simulink model "Rooms_integrated_bus13"  (R2025a)
settings: Solver=VariableStepAuto  StartTime=0.0  StopTime=5  RelTol=1e-3
libraries: spsThreePhaseVIMeasurementLib x53, fl_lib x40, nesl_utility x24, spsThreePhaseSeriesRLCLoadLib x20, spsThreePhasePISectionLineLib x20, spsLoadFlowBusLib x19, simulink x8, spsThreePhaseBreakerLib x8, spspowerguiLib x8, spsThreePhaseTransformerTwoWindingsLib x5, spsThreePhaseSourceLib x5, sps_lib x1
(part 3 of 4)

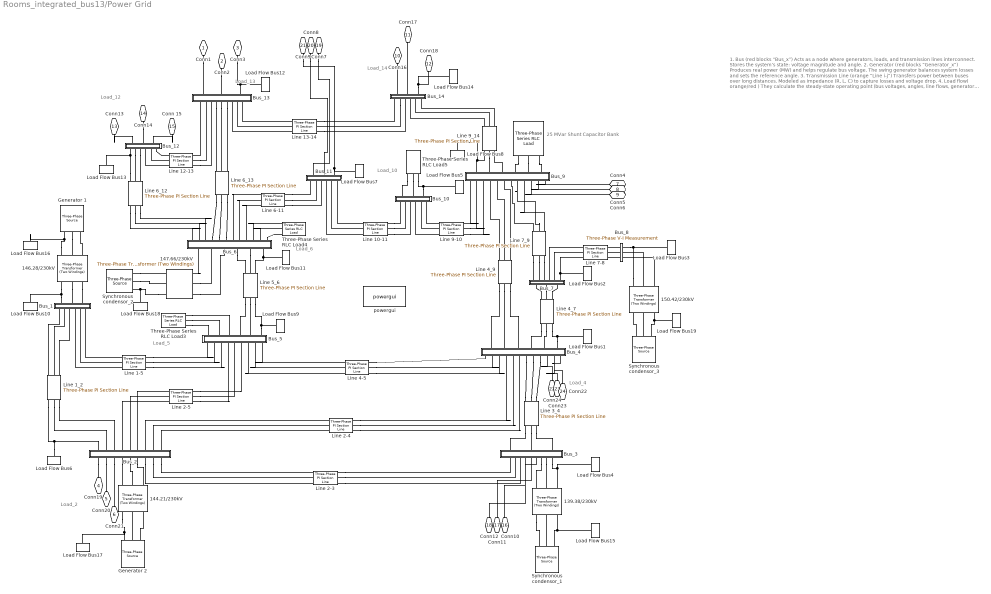
== system Rooms_integrated_bus13/Power Grid ==
  note: 1. Bus (red blocks “Bus_x”)
      | Acts as a node where generators, loads, and transmission lines interconnect.
      | Stores the system’s state: voltage magnitude and angle.
      | 2. Generator (red blocks “Generator_x”)
      | Produces real power (MW) and helps regulate bus voltage.
      | The swing generator balances system losses and sets the reference angle.
      | 3. Transmission Line (orange “Line i-j”)
      | Transfers power between buses over long distances.
      | Modeled as impedance (R, L, C) to capture losses and voltage drop.
      | 4. Load flow( orange/red )
      | They calculate the steady-state operating point (bus voltages, angles, line flows, generator outputs) before starting the simulation.
      | They provide the initial pu values (e.g., voltage magnitude & angle at each bus) so the dynamic model starts from a realistic balanced condition. .
      | 5. Synchronous Condenser (red blocks)
      | A synchronous machine running without mechanical load.
      | Supplies or absorbs reactive power to support voltage stability.
      | 6. Shunt Capacitor Bank
      | Provides fixed reactive power (Q) compensation.
      | Improves voltage profile and reduces reactive power flow in lines.
      | 7. Custom Connection Blocks (Conn1, Conn2, …)
      | Interfaces to external/custom subsystems instead of static loads.
      | Allow modeling of dynamic or special loads (e.g., EVs, converters, FACTS).
      | .
  note: Load_5
  note: Load_13
  note: Load_6
  note: Load_10
  note: Load_12
  note: Load_14
  note: Load_4
  note: 25 MVar Shunt
      | Capacitor Bank
  note: Load_2
  " " : spsThreePhaseSeriesRLCLoadLib/Three-Phase Series RLC Load  LConnTagsString=A|B|C  Configuration=Y (grounded)  NominalVoltage=230e3  Vabc=[1e3 1e3 1e3]  Vabcp=[1e3 1e3 1e3]  NominalFrequency=60  UnbalancedPower=off  ActivePower=0  InductivePower=0  CapacitivePower=25e6  Pabc=[10e3 9e3 11e3]  QLabc=[100 90 110]  QCabc=[100 90 110]  Pabcp=[10e3 9e3 11e3]  QLabcp=[100 90 110]  QCabcp=[100 90 110]  Measurements=None  LoadType=constant Z
  139.38/230kV : spsThreePhaseTransformerTwoWindingsLib/Three-Phase Transformer (Two Windings)  Winding1Connection=Yg  Winding2Connection=Yg  CoreType=Three single-phase transformers  SetSaturation=off  Hysteresis=off  DataFile='hysteresis'  SetInitialFlux=off  Measurements=None  UNITS=pu  NominalPower=[ 120e6 , 60 ]  Winding1=[139.38e3 , 0.002 , 0.08 ]  Winding2=[ 230e3 , 0.002 , 0.08 ]  Rm=500  Lm=500  L0=0.5  Saturation=[ 0,0 ; 0.0024,1.2 ; 1.0,1.52 ]  InitialFluxes=[ 0.8 , -0.8 , 0.7 ]  BreakLoop=off  DiscreteSolver=Trapezoidal iterative  DataType=off  TransfoNumber=1
  144.21/230kV : spsThreePhaseTransformerTwoWindingsLib/Three-Phase Transformer (Two Windings)  Winding1Connection=Yg  Winding2Connection=Yg  CoreType=Three single-phase transformers  SetSaturation=off  Hysteresis=off  DataFile='hysteresis'  SetInitialFlux=off  Measurements=None  UNITS=pu  NominalPower=[ 120e6 , 60 ]  Winding1=[144.21e3 , 0.002 , 0.08 ]  Winding2=[ 230e3 , 0.002 , 0.08 ]  Rm=500  Lm=500  L0=0.5  Saturation=[ 0,0 ; 0.0024,1.2 ; 1.0,1.52 ]  InitialFluxes=[ 0.8 , -0.8 , 0.7 ]  BreakLoop=off  DiscreteSolver=Trapezoidal iterative  DataType=off  TransfoNumber=1
  146.28/230kV : spsThreePhaseTransformerTwoWindingsLib/Three-Phase Transformer (Two Windings)  Winding1Connection=Yg  Winding2Connection=Yg  CoreType=Three single-phase transformers  SetSaturation=off  Hysteresis=off  DataFile='hysteresis'  SetInitialFlux=off  Measurements=None  UNITS=pu  NominalPower=[ 120e6 , 60 ]  Winding1=[146.28e3 , 0.002 , 0.08 ]  Winding2=[ 230e3 , 0.002 , 0.08 ]  Rm=500  Lm=500  L0=0.5  Saturation=[ 0,0 ; 0.0024,1.2 ; 1.0,1.52 ]  InitialFluxes=[ 0.8 , -0.8 , 0.7 ]  BreakLoop=off  DiscreteSolver=Trapezoidal iterative  DataType=off  TransfoNumber=1
  147.66/230kV : spsThreePhaseTransformerTwoWindingsLib/Three-Phase Transformer (Two Windings)  Winding1Connection=Yg  Winding2Connection=Yg  CoreType=Three single-phase transformers  SetSaturation=off  Hysteresis=off  DataFile='hysteresis'  SetInitialFlux=off  Measurements=None  UNITS=pu  NominalPower=[ 120e6 , 60 ]  Winding1=[147.66e3 , 0.002 , 0.08 ]  Winding2=[ 230e3 , 0.002 , 0.08 ]  Rm=500  Lm=500  L0=0.5  Saturation=[ 0,0 ; 0.0024,1.2 ; 1.0,1.52 ]  InitialFluxes=[ 0.8 , -0.8 , 0.7 ]  BreakLoop=off  DiscreteSolver=Trapezoidal iterative  DataType=off  TransfoNumber=1
  150.42/230kV : spsThreePhaseTransformerTwoWindingsLib/Three-Phase Transformer (Two Windings)  Winding1Connection=Yg  Winding2Connection=Yg  CoreType=Three single-phase transformers  SetSaturation=off  Hysteresis=off  DataFile='hysteresis'  SetInitialFlux=off  Measurements=None  UNITS=pu  NominalPower=[ 120e6 , 60 ]  Winding1=[150.42e3 , 0.002 , 0.08 ]  Winding2=[ 230e3 , 0.002 , 0.08 ]  Rm=500  Lm=500  L0=0.5  Saturation=[ 0,0 ; 0.0024,1.2 ; 1.0,1.52 ]  InitialFluxes=[ 0.8 , -0.8 , 0.7 ]  BreakLoop=off  DiscreteSolver=Trapezoidal iterative  DataType=off  TransfoNumber=1
  Bus_1 : Subsystem
  Bus_10 : Subsystem
  Bus_11 : Subsystem
  Bus_12 : Subsystem
  Bus_13 : Subsystem
  Bus_14 : Subsystem
  Bus_2 : Subsystem
  Bus_3 : Subsystem
  Bus_4 : Subsystem
  Bus_5 : Subsystem
  Bus_6 : Subsystem
  Bus_7 : Subsystem
  Bus_8 : spsThreePhaseVIMeasurementLib/Three-Phase V-I Measurement  VoltageMeasurement=phase-to-phase  SetLabelV=on  LabelV=VB_8  Vpu=off  VpuLL=off  CurrentMeasurement=yes  SetLabelI=on  LabelI=IB_8  Ipu=off  Pbase=100e6  Vbase=500e3  OutputType=Complex  PhasorSimulation=off  PSBequivalent=0
  Bus_9 : Subsystem
  Generator 1 : spsThreePhaseSourceLib/Three-Phase Source  InternalConnection=Yg  VoltagePhases=off  Voltage=(146280)*1.03071  PhaseAngle=3.7708  Voltage_phases=[25e3 25e3 25e3]/sqrt(3)  PhaseAngles_phases=[0 -120 +120]  Frequency=60  NonIdealSource=on  SpecifyImpedance=off  Resistance=0.8929  Inductance=16.58e-3  ShortCircuitLevel=100e6  BaseVoltage=146.28e3  XRratio=7  BusType=swing  Pref=163e6  Qref=0  Prefabc=[10e3, 10e3, 10e3]  Qrefabc=[0, 0, 0]  Qmin=-inf  Qmax=inf
  Generator 2 : spsThreePhaseSourceLib/Three-Phase Source  InternalConnection=Yg  VoltagePhases=off  Voltage=(144210)*1.01655  PhaseAngle=-15.8323  Voltage_phases=[25e3 25e3 25e3]/sqrt(3)  PhaseAngles_phases=[0 -120 +120]  Frequency=60  NonIdealSource=on  SpecifyImpedance=off  Resistance=0.8929  Inductance=16.58e-3  ShortCircuitLevel=100e6  BaseVoltage=144.21e3  XRratio=7  BusType=PV  Pref=90e6  Qref=0  Prefabc=[10e3, 10e3, 10e3]  Qrefabc=[0, 0, 0]  Qmin=-inf  Qmax=inf
  Line 1-5 : spsThreePhasePISectionLineLib/Three-Phase PI Section Line  LConnTagsString=a|b|c  RConnTagsString=A|B|C  Length=78.64  Frequency=60  Resistances=[ 0.3029 0.9086]  Inductances=[ 0.0033 0.0099]  Capacitances=[3.35e-9 1.01e-8]
  Line 10-11 : spsThreePhasePISectionLineLib/Three-Phase PI Section Line  LConnTagsString=a|b|c  RConnTagsString=A|B|C  Length=4.93  Frequency=60  Resistances=[ 0.3667 1.1002]  Inductances=[ 0.0023 0.0068]  Capacitances=[1.22e-11 3.66e-11]
  Line 12-13 : spsThreePhasePISectionLineLib/Three-Phase PI Section Line  LConnTagsString=a|b|c  RConnTagsString=A|B|C  Length=5.03  Frequency=60  Resistances=[ 0.9679 2.9038]  Inductances=[ 0.0023 0.0070]  Capacitances=[1.20e-11 3.59e-11]
  Line 13-14 : spsThreePhasePISectionLineLib/Three-Phase PI Section Line  LConnTagsString=a|b|c  RConnTagsString=A|B|C  Length=6.64  Frequency=60  Resistances=[ 0.5676 1.7027]  Inductances=[ 0.0031 0.0092]  Capacitances=[9.06e-12 2.72e-11]
  Line 1_2 : spsThreePhasePISectionLineLib/Three-Phase PI Section Line  LConnTagsString=a|b|c  RConnTagsString=A|B|C  Length=44.47  Frequency=60  Resistances=[ 0.1921 0.5763]  Inductances=[ 0.0016 0.0047]  Capacitances=[7.14e-9 2.14e-8]
  Line 2-3 : spsThreePhasePISectionLineLib/Three-Phase PI Section Line  LConnTagsString=a|b|c  RConnTagsString=A|B|C  Length=68.47  Frequency=60  Resistances=[ 0.3026 0.9077]  Inductances=[ 0.0034 0.0101]  Capacitances=[3.29e-9 9.86e-8]
  Line 2-4 : spsThreePhasePISectionLineLib/Three-Phase PI Section Line  LConnTagsString=a|b|c  RConnTagsString=A|B|C  Length=74.11  Frequency=60  Resistances=[ 0.3457 1.0370]  Inductances=[ 0.0028 0.0083]  Capacitances=[3.99e-9 1.20e-8]
  Line 2-5 : spsThreePhasePISectionLineLib/Three-Phase PI Section Line  LConnTagsString=a|b|c  RConnTagsString=A|B|C  Length=61.18  Frequency=60  Resistances=[ 0.4104 1.2311]  Inductances=[ 0.0033 0.0100]  Capacitances=[3.34e-9 1.0e-8]
  Line 3_4 : spsThreePhasePISectionLineLib/Three-Phase PI Section Line  LConnTagsString=a|b|c  RConnTagsString=A|B|C  Length=61.21  Frequency=60  Resistances=[ 0.4826 1.4479]  Inductances=[ 0.0033 0.0098]  Capacitances=[3.4e-9 1.02e-8]
  Line 4-5 : spsThreePhasePISectionLineLib/Three-Phase PI Section Line  LConnTagsString=a|b|c  RConnTagsString=A|B|C  Length=18.47  Frequency=60  Resistances=[ 0.3186 0.9558]  Inductances=[ 0.0027 0.0080]  Capacitances=[4.17e-9 1.25e-8]
  Line 4_7 : spsThreePhasePISectionLineLib/Three-Phase PI Section Line  LConnTagsString=a|b|c  RConnTagsString=A|B|C  Length=5.15  Frequency=60  Resistances=[ 0.0001 0.0003]  Inductances=[ 0.0475 0.1425]  Capacitances=[2.34e-10 7.02e-10]
  Line 4_9 : spsThreePhasePISectionLineLib/Three-Phase PI Section Line  LConnTagsString=a|b|c  RConnTagsString=A|B|C  Length=8.39  Frequency=60  Resistances=[ 0.0001 0.0003]  Inductances=[ 0.0775 0.2325]  Capacitances=[1.43e-10 4.3e-10]
  Line 5_6 : spsThreePhasePISectionLineLib/Three-Phase PI Section Line  LConnTagsString=a|b|c  RConnTagsString=A|B|C  Length=5.65  Frequency=60  Resistances=[ 0.0001 0.0003]  Inductances=[ 0.0522 0.1565]  Capacitances=[2.13e-10 6.39e-10]
  Line 6-11 : spsThreePhasePISectionLineLib/Three-Phase PI Section Line  LConnTagsString=a|b|c  RConnTagsString=A|B|C  Length=5.02  Frequency=60  Resistances=[ 0.4172 1.2515]  Inductances=[ 0.0023 0.0070]  Capacitances=[1.20e-11 3.60e-11]
  Line 6_12 : spsThreePhasePISectionLineLib/Three-Phase PI Section Line  LConnTagsString=a|b|c  RConnTagsString=A|B|C  Length=5.69  Frequency=60  Resistances=[ 0.4760 1.4281]  Inductances=[ 0.0026 0.0079]  Capacitances=[1.06e-11 3.17e-11]
  Line 6_13 : spsThreePhasePISectionLineLib/Three-Phase PI Section Line  LConnTagsString=a|b|c  RConnTagsString=A|B|C  Length=4.06  Frequency=60  Resistances=[ 0.3590 1.0770]  Inductances=[ 0.0019 0.0056]  Capacitances=[1.48e-11 4.44e-11]
  Line 7-8 : spsThreePhasePISectionLineLib/Three-Phase PI Section Line  LConnTagsString=a|b|c  RConnTagsString=A|B|C  Length=4.72  Frequency=60  Resistances=[ 0.0005 0.0014]  Inductances=[ 0.0022 0.0065]  Capacitances=[ 1.27e-11 3.82e-11]
  Line 7_9 : spsThreePhasePISectionLineLib/Three-Phase PI Section Line  LConnTagsString=a|b|c  RConnTagsString=A|B|C  Length=3.73  Frequency=60  Resistances=[ 0.0006 0.0018]  Inductances=[ 0.0017 0.0052]  Capacitances=[ 1.61e-11 4.84e-11]
  Line 9-10 : spsThreePhasePISectionLineLib/Three-Phase PI Section Line  LConnTagsString=a|b|c  RConnTagsString=A|B|C  Length=3.27  Frequency=60  Resistances=[ 0.2144 0.6431]  Inductances=[ 0.0015 0.0045]  Capacitances=[1.84e-11 5.52e-11]
  Line 9_14 : spsThreePhasePISectionLineLib/Three-Phase PI Section Line  LConnTagsString=a|b|c  RConnTagsString=A|B|C  Length=5.85  Frequency=60  Resistances=[ 0.4788 1.4365]  Inductances=[ 0.0027 0.0081]  Capacitances=[1.03e-11 3.08e-11]
  Load Flow Bus1 : spsLoadFlowBusLib/Load Flow Bus  LConnTagsString=a  Phases=single  Connectors=on one side  ID=BUS_4  Vbase=230e3  Vref=1  Vangle=0  VLF=0.928  VLFb=1  VLFc=1  angleLF=-31.28  angleLFb=0  angleLFc=0
  Load Flow Bus10 : spsLoadFlowBusLib/Load Flow Bus  LConnTagsString=a  Phases=single  Connectors=on one side  ID=BUS_1  Vbase=230e3  Vref=1.0  Vangle=0  VLF=0.9625  VLFb=1  VLFc=1  angleLF=-19.37  angleLFb=0  angleLFc=0
  Load Flow Bus11 : spsLoadFlowBusLib/Load Flow Bus  LConnTagsString=a  Phases=single  Connectors=on one side  ID=BUS_6  Vbase=230e3  Vref=1  Vangle=0  VLF=0.9425  VLFb=1  VLFc=1  angleLF=-36.08  angleLFb=0  angleLFc=0
  Load Flow Bus12 : spsLoadFlowBusLib/Load Flow Bus  LConnTagsString=a  Phases=single  Connectors=on one side  ID=BUS_13  Vbase=230e3  Vref=1  Vangle=0  VLF=0.9416  VLFb=1  VLFc=1  angleLF=-36.14  angleLFb=0  angleLFc=0
  Load Flow Bus13 : spsLoadFlowBusLib/Load Flow Bus  LConnTagsString=a  Phases=single  Connectors=on one side  ID=BUS_12  Vbase=230e3  Vref=1.0  Vangle=0  VLF=0.9418  VLFb=1  VLFc=1  angleLF=-36.13  angleLFb=0  angleLFc=0
  Load Flow Bus14 : spsLoadFlowBusLib/Load Flow Bus  LConnTagsString=a  Phases=single  Connectors=on one side  ID=BUS_14  Vbase=230e3  Vref=1  Vangle=0  VLF=0.9414  VLFb=1  VLFc=1  angleLF=-36.19  angleLFb=0  angleLFc=0
  Load Flow Bus15 : spsLoadFlowBusLib/Load Flow Bus  LConnTagsString=a  Phases=single  Connectors=on one side  ID=BUS_c  Vbase=139.38e3  Vref=1  Vangle=0  VLF=0.9282  VLFb=1  VLFc=1  angleLF=-34.24  angleLFb=0  angleLFc=0
  Load Flow Bus16 : spsLoadFlowBusLib/Load Flow Bus  LConnTagsString=a  Phases=single  Connectors=on one side  ID=BUS_a  Vbase=146.28e3  Vref=1.0  Vangle=0  VLF=0.9625  VLFb=1  VLFc=1  angleLF=-19.37  angleLFb=0  angleLFc=0
  Load Flow Bus17 : spsLoadFlowBusLib/Load Flow Bus  LConnTagsString=a  Phases=single  Connectors=on one side  ID=BUS_b  Vbase=144.21e3  Vref=1.025  Vangle=0  VLF=0.9497  VLFb=1  VLFc=1  angleLF=-24.42  angleLFb=0  angleLFc=0
  Load Flow Bus18 : spsLoadFlowBusLib/Load Flow Bus  LConnTagsString=a  Phases=single  Connectors=on one side  ID=BUS_d  Vbase=147.66e3  Vref=1.0  Vangle=0  VLF=0.9625  VLFb=1  VLFc=1  angleLF=-19.37  angleLFb=0  angleLFc=0
  Load Flow Bus19 : spsLoadFlowBusLib/Load Flow Bus  LConnTagsString=a  Phases=single  Connectors=on one side  ID=BUS_e  Vbase=150.420e3  Vref=1  Vangle=0  VLF=0.9461  VLFb=1  VLFc=1  angleLF=-36  angleLFb=0  angleLFc=0
  Load Flow Bus2 : spsLoadFlowBusLib/Load Flow Bus  LConnTagsString=a  Phases=single  Connectors=on one side  ID=BUS_7  Vbase=230e3  Vref=1  Vangle=0  VLF=0.9439  VLFb=1  VLFc=1  angleLF=-36  angleLFb=0  angleLFc=0
  Load Flow Bus3 : spsLoadFlowBusLib/Load Flow Bus  LConnTagsString=a  Phases=single  Connectors=on one side  ID=BUS_8  Vbase=230e3  Vref=1  Vangle=0  VLF=0.9461  VLFb=1  VLFc=1  angleLF=-36  angleLFb=0  angleLFc=0
  Load Flow Bus4 : spsLoadFlowBusLib/Load Flow Bus  LConnTagsString=a  Phases=single  Connectors=on one side  ID=BUS_3  Vbase=230e3  Vref=1  Vangle=0  VLF=0.9282  VLFb=1  VLFc=1  angleLF=-34.24  angleLFb=0  angleLFc=0
  Load Flow Bus5 : spsLoadFlowBusLib/Load Flow Bus  LConnTagsString=a  Phases=single  Connectors=on one side  ID=BUS_10  Vbase=230e3  Vref=1  Vangle=0  VLF=0.9425  VLFb=1  VLFc=1  angleLF=-36.13  angleLFb=0  angleLFc=0
  Load Flow Bus6 : spsLoadFlowBusLib/Load Flow Bus  LConnTagsString=a  Phases=single  Connectors=on one side  ID=BUS_2  Vbase=230e3  Vref=1.0  Vangle=0  VLF=0.9497  VLFb=1  VLFc=1  angleLF=-24.42  angleLFb=0  angleLFc=0
  Load Flow Bus7 : spsLoadFlowBusLib/Load Flow Bus  LConnTagsString=a  Phases=single  Connectors=on one side  ID=BUS_11  Vbase=230e3  Vref=1  Vangle=0  VLF=0.9423  VLFb=1  VLFc=1  angleLF=-36.11  angleLFb=0  angleLFc=0
  Load Flow Bus8 : spsLoadFlowBusLib/Load Flow Bus  LConnTagsString=a  Phases=single  Connectors=on one side  ID=BUS_9  Vbase=230e3  Vref=1.0  Vangle=0  VLF=0.943  VLFb=1  VLFc=1  angleLF=-36.12  angleLFb=0  angleLFc=0
  Load Flow Bus9 : spsLoadFlowBusLib/Load Flow Bus  LConnTagsString=a  Phases=single  Connectors=on one side  ID=BUS_5  Vbase=230e3  Vref=1  Vangle=0  VLF=0.9312  VLFb=1  VLFc=1  angleLF=-29.41  angleLFb=0  angleLFc=0
  Synchronous condensor_1 : spsThreePhaseSourceLib/Three-Phase Source  InternalConnection=Yg  VoltagePhases=off  Voltage=(139380)*1.01137  PhaseAngle=-34.48  Voltage_phases=[25e3 25e3 25e3]/sqrt(3)  PhaseAngles_phases=[0 -120 +120]  Frequency=60  NonIdealSource=on  SpecifyImpedance=off  Resistance=0.8929  Inductance=16.58e-3  ShortCircuitLevel=100e6  BaseVoltage=139.38e3  XRratio=7  BusType=PQ  Pref=0  Qref=50.096e6  Prefabc=[10e3, 10e3, 10e3]  Qrefabc=[0, 0, 0]  Qmin=-inf  Qmax=inf
  Synchronous condensor_2 : spsThreePhaseSourceLib/Three-Phase Source  InternalConnection=Yg  VoltagePhases=off  Voltage=(147660)*0.984306  PhaseAngle=-36.2022  Voltage_phases=[25e3 25e3 25e3]/sqrt(3)  PhaseAngles_phases=[0 -120 +120]  Frequency=60  NonIdealSource=on  SpecifyImpedance=off  Resistance=0.8929  Inductance=16.58e-3  ShortCircuitLevel=100e6  BaseVoltage=147.66e3  XRratio=7  BusType=PQ  Pref=0  Qref=25.276e6  Prefabc=[10e3, 10e3, 10e3]  Qrefabc=[0, 0, 0]  Qmin=-inf  Qmax=inf
  Synchronous condensor_3 : spsThreePhaseSourceLib/Three-Phase Source  InternalConnection=Yg  VoltagePhases=off  Voltage=(150420)*0.995122  PhaseAngle=-36.1424  Voltage_phases=[25e3 25e3 25e3]/sqrt(3)  PhaseAngles_phases=[0 -120 +120]  Frequency=60  NonIdealSource=on  SpecifyImpedance=off  Resistance=0.8929  Inductance=16.58e-3  ShortCircuitLevel=100e6  BaseVoltage=150.42e3  XRratio=7  BusType=PQ  Pref=0  Qref=30.144e6  Prefabc=[10e3, 10e3, 10e3]  Qrefabc=[0, 0, 0]  Qmin=-inf  Qmax=inf
  Three-Phase Series RLC Load3 : spsThreePhaseSeriesRLCLoadLib/Three-Phase Series RLC Load  LConnTagsString=A|B|C  Configuration=Y (grounded)  NominalVoltage=(230000)*0.931217  Vabc=[1e3 1e3 1e3]  Vabcp=[1e3 1e3 1e3]  NominalFrequency=60  UnbalancedPower=off  ActivePower=9.12e6  InductivePower=1.92e6  CapacitivePower=0  Pabc=[10e3 9e3 11e3]  QLabc=[100 90 110]  QCabc=[100 90 110]  Pabcp=[10e3 9e3 11e3]  QLabcp=[100 90 110]  QCabcp=[100 90 110]  Measurements=None  LoadType=constant PQ
  Three-Phase Series RLC Load4 : spsThreePhaseSeriesRLCLoadLib/Three-Phase Series RLC Load  LConnTagsString=A|B|C  Configuration=Y (grounded)  NominalVoltage=(230000)*0.942548  Vabc=[1e3 1e3 1e3]  Vabcp=[1e3 1e3 1e3]  NominalFrequency=60  UnbalancedPower=off  ActivePower=13.44e6  InductivePower=9e6  CapacitivePower=0  Pabc=[10e3 9e3 11e3]  QLabc=[100 90 110]  QCabc=[100 90 110]  Pabcp=[10e3 9e3 11e3]  QLabcp=[100 90 110]  QCabcp=[100 90 110]  Measurements=None  LoadType=constant PQ
  Three-Phase Series RLC Load5 : spsThreePhaseSeriesRLCLoadLib/Three-Phase Series RLC Load  LConnTagsString=A|B|C  Configuration=Y (grounded)  NominalVoltage=(230000)*0.942502  Vabc=[1e3 1e3 1e3]  Vabcp=[1e3 1e3 1e3]  NominalFrequency=60  UnbalancedPower=off  ActivePower=10.8e6  InductivePower=6.96e6  CapacitivePower=0  Pabc=[10e3 9e3 11e3]  QLabc=[100 90 110]  QCabc=[100 90 110]  Pabcp=[10e3 9e3 11e3]  QLabcp=[100 90 110]  QCabcp=[100 90 110]  Measurements=None  LoadType=constant PQ
  powergui : spspowerguiLib/powergui  Priority=1  SimulationMode=Discrete  SampleTime=50e-6  frequency=60  Iterations=50  frequencyindice=60  Pbase=120e6  ErrMax=0.0001  UnitsV=kV  UnitsW=MW  buscounter=0  FunctionMessages=off  echomessages=off  EnableUseOfTLC=off  CurrentSourceSwitches=off  DisableSnubberDevices=off  DisableRonSwitches=off  DisableVfSwitches=off  DisplayEquations=off  AutomaticDiscreteSolvers=off  SolverType=Tustin/Backward Euler (TBE)  Interpol=off  ExternalGateDelay=off  methode=off  Ts=100  x0status=blocks  SPID=on  SwTol=0  HookPort=off  NonlinearTolerance=1e-4  nMaxIteration=100  ContinueOnMaxIteration=off  RestoreLinks=warning  ResistiveCurrentMeasurement=off  Frange=[0:2:500]  Ylog=off  Xlog=on  ShowGrid=off  save=off  variable=ZData  structure=0  ZoomFFT=off  StartTime=0.0  cycles=1  DisplayStyle=1  fundamental=60  FreqAxis=off  MaxFrequency=1000  frequencyindicesteady=1  RmsSteady=1  display=off
  Conn1 : PMIOPort  Side=Left
  Conn2 : PMIOPort  Port=2  Side=Left
  Conn3 : PMIOPort  Port=3  Side=Left
  Conn19 : PMIOPort  Port=4  Side=Left
  Conn20 : PMIOPort  Port=5  Side=Left
  Conn21 : PMIOPort  Port=6  Side=Left
  Conn4 : PMIOPort  Port=7  Side=Left
  Conn5 : PMIOPort  Port=8  Side=Left
  Conn6 : PMIOPort  Port=9  Side=Left
  Conn16 : PMIOPort  Port=10  Side=Left
  Conn17 : PMIOPort  Port=11  Side=Left
  Conn18 : PMIOPort  Port=12  Side=Left
  Conn13 : PMIOPort  Port=13  Side=Right
  Conn14 : PMIOPort  Port=14  Side=Right
  Conn 15 : PMIOPort  Port=15  Side=Right
  Conn10 : PMIOPort  Port=16  Side=Right
  Conn11 : PMIOPort  Port=17  Side=Right
  Conn12 : PMIOPort  Port=18  Side=Right
  Conn7 : PMIOPort  Port=19  Side=Right
  Conn8 : PMIOPort  Port=20  Side=Right
  Conn9 : PMIOPort  Port=21  Side=Right
  Conn24 : PMIOPort  Port=22  Side=Right
  Conn23 : PMIOPort  Port=23  Side=Right
  Conn22 : PMIOPort  Port=24  Side=Right
  connections:
  Synchronous condensor_3/RConn1 -- 150.42/230kV/LConn1
  Bus_2/RConn4 -- 144.21/230kV/RConn1
  Line 10-11/LConn1 -- Bus_11/RConn6
  Line 6_12/RConn1 -- Bus_6/RConn1
  147.66/230kV/LConn3 -- Synchronous condensor_2/RConn3 -- Load Flow Bus18/LConn1
  Line 2-5/RConn3 -- Bus_5/RConn4
  Conn7/RConn1 -- Bus_11/LConn1
  Line 9_14/RConn1 -- Bus_9/LConn1 -- Load Flow Bus8/LConn1
  Bus_4/RConn7 -- Line 3_4/LConn1
  146.28/230kV/RConn1 -- Bus_1/LConn3
  Line 12-13/RConn3 -- Bus_13/RConn3
  Line 9-10/LConn3 -- Bus_10/RConn4
  Line 2-5/RConn2 -- Bus_5/RConn5
  Generator 2/RConn1 -- 144.21/230kV/LConn1 -- Load Flow Bus17/LConn1
  Line 4_9/RConn1 -- Bus_4/LConn1
  Bus_2/LConn5 -- Line 2-5/LConn2
  Load Flow Bus12/LConn1 -- Conn3/RConn1 -- Bus_13/LConn3
  Bus_5/LConn6 -- Line 5_6/RConn3 -- Load Flow Bus9/LConn1
  Load Flow Bus11/LConn1 -- Bus_6/LConn6 -- Line 5_6/LConn3
  Bus_11/LConn3 -- Conn9/RConn1 -- Load Flow Bus7/LConn1
  147.66/230kV/RConn3 -- Bus_6/LConn3
  Line 4_7/RConn1 -- Bus_4/LConn4
  Line 4-5/RConn1 -- Bus_4/RConn1
  Bus_6/LConn5 -- Line 5_6/LConn2
  Bus_14/LConn3 -- Conn18/RConn1 -- Load Flow Bus14/LConn1
  Line 9-10/RConn2 -- Bus_9/RConn2
  Line 6-11/RConn2 -- Bus_11/RConn2
  Line 4-5/LConn2 -- Bus_5/RConn8
  Bus_2/RConn1 -- Conn19/RConn1
  Line 6-11/LConn2 -- Bus_6/RConn8
  Line 2-3/RConn1 -- Bus_3/RConn1
  150.42/230kV/LConn3 -- Synchronous condensor_3/RConn3 -- Load Flow Bus19/LConn1
  Load Flow Bus15/LConn1 -- Synchronous condensor_1/RConn3 -- 139.38/230kV/LConn3
  Line 7_9/LConn3 -- Bus_9/RConn9
  Line 9_14/RConn2 -- Bus_9/LConn2
  Bus_7/RConn6 -- Line 7-8/LConn3 -- Load Flow Bus2/LConn1
  Bus_2/RConn3 -- Conn21/RConn1
  Line 4-5/RConn3 -- Bus_4/RConn3
  Line 4_9/LConn1 -- Bus_9/RConn4
  150.42/230kV/RConn1 -- Bus_8/RConn1 -- Load Flow Bus3/LConn1
  Line 7-8/LConn1 -- Bus_7/RConn4
  Line 1_2/RConn2 -- Bus_2/LConn2
  Line 1-5/RConn1 -- Bus_5/RConn1
  Bus_4/LConn6 -- Line 4_7/RConn3 -- Load Flow Bus1/LConn1
  Line 6_12/LConn1 -- Bus_12/RConn1 -- Load Flow Bus13/LConn1
  Line 6-11/LConn3 -- Bus_6/RConn9
  Load Flow Bus4/LConn1 -- Bus_3/RConn9 -- 139.38/230kV/RConn3
  146.28/230kV/LConn3 -- Generator 1/RConn3 -- Load Flow Bus16/LConn1
  Line 1_2/LConn1 -- Bus_1/RConn1
  Bus_13/RConn6 -- Line 6_13/LConn3
  Load Flow Bus6/LConn1 -- Line 1_2/RConn1 -- Bus_2/LConn1
  Line 1-5/RConn2 -- Bus_5/RConn2
  Line 2-4/LConn3 -- Bus_2/LConn9
  Bus_10/LConn3 -- Load Flow Bus5/LConn1 -- Three-Phase Series RLC Load5/LConn3
  Conn10/RConn1 -- Bus_3/RConn4
  Line 6-11/RConn1 -- Bus_11/RConn1
  Bus_8/LConn2 -- Line 7-8/RConn2
  Line 9_14/LConn3 -- Bus_14/RConn6
  Line 10-11/LConn2 -- Bus_11/RConn5
  Generator 2/RConn2 -- 144.21/230kV/LConn2
  Bus_1/LConn1 -- 146.28/230kV/RConn3 -- Load Flow Bus10/LConn1
  146.28/230kV/RConn2 -- Bus_1/LConn2
  Line 13-14/RConn3 -- Bus_14/RConn3
  139.38/230kV/LConn1 -- Synchronous condensor_1/RConn1
  Line 10-11/RConn1 -- Bus_10/RConn1
  Line 7_9/LConn2 -- Bus_9/RConn8
  Line 4_7/LConn3 -- Bus_7/LConn3
  Three-Phase Series RLC Load4/LConn1 -- Bus_6/RConn10
  150.42/230kV/RConn2 -- Bus_8/RConn2
  Line 3_4/RConn1 -- Bus_3/LConn1
  Line 3_4/RConn3 -- Bus_3/LConn3
  Conn24/RConn1 -- Bus_4/RConn10
  Line 1_2/LConn3 -- Bus_1/RConn3
  Synchronous condensor_2/RConn2 -- 147.66/230kV/LConn2
  Bus_2/RConn6 -- 144.21/230kV/RConn3
  Line 12-13/LConn2 -- Bus_12/RConn5
  Line 4_9/RConn3 -- Bus_4/LConn3
  Bus_13/RConn5 -- Line 6_13/LConn2
  Synchronous condensor_1/RConn2 -- 139.38/230kV/LConn2
  Line 9-10/RConn3 -- Bus_9/RConn3
  Line 1-5/LConn2 -- Bus_1/RConn5
  Line 4-5/LConn3 -- Bus_5/RConn7
  Line 5_6/RConn2 -- Bus_5/LConn5
  Line 13-14/LConn1 -- Bus_13/RConn9
  Line 9_14/LConn1 -- Bus_14/RConn4
  Bus_12/RConn2 -- Line 6_12/LConn2
  Three-Phase Series RLC Load5/LConn1 -- Bus_10/LConn1
  Line 6_13/RConn1 -- Bus_6/RConn4
  Line 12-13/RConn1 -- Bus_13/RConn1
  Three-Phase Series RLC Load3/LConn3 -- Bus_5/LConn1
  Line 6_12/RConn3 -- Bus_6/RConn3
  Line 1_2/RConn3 -- Bus_2/LConn3
  Line 4_7/RConn2 -- Bus_4/LConn5
  Line 7_9/RConn1 -- Bus_7/RConn1
  Generator 2/RConn3 -- 144.21/230kV/LConn3
  Generator 1/RConn2 -- 146.28/230kV/LConn2
  Line 2-3/RConn3 -- Bus_3/RConn3
  Bus_12/RConn3 -- Line 6_12/LConn3
  Conn1/RConn1 -- Bus_13/LConn1
  Line 6-11/RConn3 -- Bus_11/RConn3
  Line 13-14/LConn2 -- Bus_13/RConn8
  150.42/230kV/RConn3 -- Bus_8/RConn3
  Line 4_9/LConn3 -- Bus_9/RConn6
  Conn14/RConn1 -- Bus_12/LConn2
  Bus_8/LConn1 -- Line 7-8/RConn1
  Line 7-8/LConn2 -- Bus_7/RConn5
  Line 12-13/LConn1 -- Bus_12/RConn6
  Line 7_9/RConn3 -- Bus_7/RConn3
  Line 2-4/LConn1 -- Bus_2/LConn7
  Line 5_6/RConn1 -- Bus_5/LConn4
  Synchronous condensor_3/RConn2 -- 150.42/230kV/LConn2
  Bus_2/RConn2 -- Conn20/RConn1
  Line 1-5/LConn1 -- Bus_1/RConn6
  Line 10-11/RConn3 -- Bus_10/RConn3
  Three-Phase Series RLC Load5/LConn2 -- Bus_10/LConn2
  Line 13-14/LConn3 -- Bus_13/RConn7
  Bus_14/LConn2 -- Conn17/RConn1
  Three-Phase Series RLC Load3/LConn1 -- Bus_5/LConn3
  Bus_6/LConn4 -- Line 5_6/LConn1
  Bus_2/RConn5 -- 144.21/230kV/RConn2
  Conn5/RConn1 -- Bus_9/RConn11
  Line 10-11/RConn2 -- Bus_10/RConn2
  Three-Phase Series RLC Load4/LConn2 -- Bus_6/RConn11
  Line 1-5/RConn3 -- Bus_5/RConn3
  Line 2-5/LConn3 -- Bus_2/LConn4
  " "/LConn3 -- Bus_9/LConn6
  Line 13-14/RConn1 -- Bus_14/RConn1
  Bus_2/RConn7 -- Line 2-3/LConn3
  Bus_3/RConn7 -- 139.38/230kV/RConn1
  Conn22/RConn1 -- Bus_4/RConn12
  Line 7_9/RConn2 -- Bus_7/RConn2
  Conn4/RConn1 -- Bus_9/RConn12
  Bus_13/RConn4 -- Line 6_13/LConn1
  Line 6_13/RConn3 -- Bus_6/RConn6
  Bus_2/RConn8 -- Line 2-3/LConn2
  Bus_4/RConn8 -- Line 3_4/LConn2
  Bus_2/RConn9 -- Line 2-3/LConn1
  Conn13/RConn1 -- Bus_12/LConn1
  Conn 15/RConn1 -- Bus_12/LConn3
  Line 9_14/LConn2 -- Bus_14/RConn5
  Line 3_4/RConn2 -- Bus_3/LConn2
  Line 6_13/RConn2 -- Bus_6/RConn5
  Line 6-11/LConn1 -- Bus_6/RConn7
  Line 12-13/LConn3 -- Bus_12/RConn4
  Three-Phase Series RLC Load3/LConn2 -- Bus_5/LConn2
  Line 12-13/RConn2 -- Bus_13/RConn2
  Bus_9/LConn3 -- Line 9_14/RConn3
  Line 4_7/LConn1 -- Bus_7/LConn1
  Line 2-4/LConn2 -- Bus_2/LConn8
  Line 2-3/RConn2 -- Bus_3/RConn2
  Three-Phase Series RLC Load4/LConn3 -- Bus_6/RConn12
  147.66/230kV/RConn1 -- Bus_6/LConn1
  Conn23/RConn1 -- Bus_4/RConn11
  Bus_8/LConn3 -- Line 7-8/RConn3
  Line 7_9/LConn1 -- Bus_9/RConn7
  146.28/230kV/LConn1 -- Generator 1/RConn1
  147.66/230kV/RConn2 -- Bus_6/LConn2
  Line 9-10/RConn1 -- Bus_9/RConn1
  Line 4_9/LConn2 -- Bus_9/RConn5
  Line 2-4/RConn1 -- Bus_4/RConn4
  Line 4_9/RConn2 -- Bus_4/LConn2
  Line 4-5/LConn1 -- Bus_5/RConn9
  Line 2-4/RConn3 -- Bus_4/RConn6
  Bus_7/LConn2 -- Line 4_7/LConn2
  Synchronous condensor_2/RConn1 -- 147.66/230kV/LConn1
  Line 9-10/LConn2 -- Bus_10/RConn5
  Bus_14/LConn1 -- Conn16/RConn1
  " "/LConn1 -- Bus_9/LConn4
  Line 2-5/RConn1 -- Bus_5/RConn6
  Line 1-5/LConn3 -- Bus_1/RConn4
  Line 10-11/LConn3 -- Bus_11/RConn4
  Line 9-10/LConn1 -- Bus_10/RConn6
  " "/LConn2 -- Bus_9/LConn5
  Line 6_12/RConn2 -- Bus_6/RConn2
  Line 1_2/LConn2 -- Bus_1/RConn2
  Line 2-5/LConn1 -- Bus_2/LConn6
  Line 4-5/RConn2 -- Bus_4/RConn2
  Line 2-4/RConn2 -- Bus_4/RConn5
  Bus_14/RConn2 -- Line 13-14/RConn2
  Bus_3/RConn8 -- 139.38/230kV/RConn2
  Bus_4/RConn9 -- Line 3_4/LConn3
  Conn2/RConn1 -- Bus_13/LConn2
  Conn8/RConn1 -- Bus_11/LConn2
  Conn11/RConn1 -- Bus_3/RConn5
  Conn12/RConn1 -- Bus_3/RConn6
  Conn6/RConn1 -- Bus_9/RConn10

== system Rooms_integrated_bus13/Power Grid/Bus_1 ==
  Bus : spsThreePhaseVIMeasurementLib/Three-Phase V-I Measurement  VoltageMeasurement=phase-to-phase  SetLabelV=on  LabelV=VB_1  Vpu=off  VpuLL=off  CurrentMeasurement=yes  SetLabelI=on  LabelI=IB_1  Ipu=off  Pbase=100e6  Vbase=500e3  OutputType=Complex  PhasorSimulation=off  PSBequivalent=0
  Bus_ : spsThreePhaseVIMeasurementLib/Three-Phase V-I Measurement  VoltageMeasurement=phase-to-phase  SetLabelV=on  LabelV=V_B1  Vpu=off  VpuLL=off  CurrentMeasurement=yes  SetLabelI=on  LabelI=I_B1  Ipu=off  Pbase=100e6  Vbase=500e3  OutputType=Complex  PhasorSimulation=off  PSBequivalent=0
  Conn1 : PMIOPort  Side=Left
  Conn2 : PMIOPort  Port=2  Side=Right
  Conn3 : PMIOPort  Port=3  Side=Left
  Conn4 : PMIOPort  Port=4  Side=Right
  Conn5 : PMIOPort  Port=5  Side=Right
  Conn6 : PMIOPort  Port=6  Side=Left
  Conn7 : PMIOPort  Port=7  Side=Right
  Conn8 : PMIOPort  Port=8  Side=Right
  Conn9 : PMIOPort  Port=9  Side=Right
  connections:
  Conn6/RConn1 -- Bus_/LConn1 -- Bus/LConn3
  Bus/RConn2 -- Conn4/RConn1
  Bus_/RConn2 -- Conn8/RConn1
  Bus/LConn2 -- Bus_/LConn2 -- Conn3/RConn1
  Bus/LConn1 -- Bus_/LConn3 -- Conn1/RConn1
  Conn5/RConn1 -- Bus/RConn1
  Conn2/RConn1 -- Bus/RConn3
  Conn9/RConn1 -- Bus_/RConn1
  Conn7/RConn1 -- Bus_/RConn3

== system Rooms_integrated_bus13/Power Grid/Bus_10 ==
  Bus : spsThreePhaseVIMeasurementLib/Three-Phase V-I Measurement  VoltageMeasurement=phase-to-phase  SetLabelV=on  LabelV=VB_10  Vpu=off  VpuLL=off  CurrentMeasurement=yes  SetLabelI=on  LabelI=IB_10  Ipu=off  Pbase=100e6  Vbase=500e3  OutputType=Complex  PhasorSimulation=off  PSBequivalent=0
  Bus_ : spsThreePhaseVIMeasurementLib/Three-Phase V-I Measurement  VoltageMeasurement=phase-to-phase  SetLabelV=on  LabelV=V_B10  Vpu=off  VpuLL=off  CurrentMeasurement=yes  SetLabelI=on  LabelI=I_B10  Ipu=off  Pbase=100e6  Vbase=500e3  OutputType=Complex  PhasorSimulation=off  PSBequivalent=0
  Conn1 : PMIOPort  Side=Left
  Conn2 : PMIOPort  Port=2  Side=Right
  Conn3 : PMIOPort  Port=3  Side=Left
  Conn4 : PMIOPort  Port=4  Side=Right
  Conn5 : PMIOPort  Port=5  Side=Right
  Conn6 : PMIOPort  Port=6  Side=Left
  Conn7 : PMIOPort  Port=7  Side=Right
  Conn8 : PMIOPort  Port=8  Side=Right
  Conn9 : PMIOPort  Port=9  Side=Right
  connections:
  Conn1/RConn1 -- Bus_/LConn3 -- Bus/LConn1
  Conn3/RConn1 -- Bus_/LConn2 -- Bus/LConn2
  Bus_/RConn2 -- Conn8/RConn1
  Bus/RConn2 -- Conn4/RConn1
  Bus/LConn3 -- Bus_/LConn1 -- Conn6/RConn1
  Bus_/RConn1 -- Conn7/RConn1
  Bus_/RConn3 -- Conn9/RConn1
  Bus/RConn1 -- Conn2/RConn1
  Bus/RConn3 -- Conn5/RConn1

== system Rooms_integrated_bus13/Power Grid/Bus_11 ==
  Bus : spsThreePhaseVIMeasurementLib/Three-Phase V-I Measurement  VoltageMeasurement=phase-to-phase  SetLabelV=on  LabelV=VB_11  Vpu=off  VpuLL=off  CurrentMeasurement=yes  SetLabelI=on  LabelI=IB_11  Ipu=off  Pbase=100e6  Vbase=500e3  OutputType=Complex  PhasorSimulation=off  PSBequivalent=0
  Bus_ : spsThreePhaseVIMeasurementLib/Three-Phase V-I Measurement  VoltageMeasurement=phase-to-phase  SetLabelV=on  LabelV=V_B11  Vpu=off  VpuLL=off  CurrentMeasurement=yes  SetLabelI=on  LabelI=I_B11  Ipu=off  Pbase=100e6  Vbase=500e3  OutputType=Complex  PhasorSimulation=off  PSBequivalent=0
  Conn1 : PMIOPort  Side=Left
  Conn2 : PMIOPort  Port=2  Side=Right
  Conn3 : PMIOPort  Port=3  Side=Left
  Conn4 : PMIOPort  Port=4  Side=Right
  Conn5 : PMIOPort  Port=5  Side=Right
  Conn6 : PMIOPort  Port=6  Side=Left
  Conn7 : PMIOPort  Port=7  Side=Right
  Conn8 : PMIOPort  Port=8  Side=Right
  Conn9 : PMIOPort  Port=9  Side=Right
  connections:
  Bus/RConn3 -- Conn5/RConn1
  Bus/RConn1 -- Conn2/RConn1
  Bus_/RConn3 -- Conn9/RConn1
  Bus_/RConn1 -- Conn7/RConn1
  Conn6/RConn1 -- Bus_/LConn1 -- Bus/LConn3
  Bus/RConn2 -- Conn4/RConn1
  Bus_/RConn2 -- Conn8/RConn1
  Bus/LConn2 -- Bus_/LConn2 -- Conn3/RConn1
  Bus/LConn1 -- Conn1/RConn1 -- Bus_/LConn3

== system Rooms_integrated_bus13/Power Grid/Bus_12 ==
  Bus : spsThreePhaseVIMeasurementLib/Three-Phase V-I Measurement  VoltageMeasurement=phase-to-phase  SetLabelV=on  LabelV=VB_12  Vpu=off  VpuLL=off  CurrentMeasurement=yes  SetLabelI=on  LabelI=IB_12  Ipu=off  Pbase=100e6  Vbase=500e3  OutputType=Complex  PhasorSimulation=off  PSBequivalent=0
  Bus_ : spsThreePhaseVIMeasurementLib/Three-Phase V-I Measurement  VoltageMeasurement=phase-to-phase  SetLabelV=on  LabelV=V_B12  Vpu=off  VpuLL=off  CurrentMeasurement=yes  SetLabelI=on  LabelI=I_B12  Ipu=off  Pbase=100e6  Vbase=500e3  OutputType=Complex  PhasorSimulation=off  PSBequivalent=0
  Conn1 : PMIOPort  Side=Left
  Conn2 : PMIOPort  Port=2  Side=Right
  Conn3 : PMIOPort  Port=3  Side=Left
  Conn4 : PMIOPort  Port=4  Side=Right
  Conn5 : PMIOPort  Port=5  Side=Right
  Conn6 : PMIOPort  Port=6  Side=Left
  Conn7 : PMIOPort  Port=7  Side=Right
  Conn8 : PMIOPort  Port=8  Side=Right
  Conn9 : PMIOPort  Port=9  Side=Right
  connections:
  Conn1/RConn1 -- Bus_/LConn3 -- Bus/LConn1
  Conn3/RConn1 -- Bus_/LConn2 -- Bus/LConn2
  Bus_/RConn2 -- Conn8/RConn1
  Bus/RConn2 -- Conn4/RConn1
  Bus/LConn3 -- Bus_/LConn1 -- Conn6/RConn1
  Bus_/RConn1 -- Conn7/RConn1
  Bus_/RConn3 -- Conn9/RConn1
  Bus/RConn1 -- Conn2/RConn1
  Bus/RConn3 -- Conn5/RConn1

== system Rooms_integrated_bus13/Power Grid/Bus_13 ==
  Bus : spsThreePhaseVIMeasurementLib/Three-Phase V-I Measurement  VoltageMeasurement=phase-to-phase  SetLabelV=on  LabelV=VB_13  Vpu=off  VpuLL=off  CurrentMeasurement=yes  SetLabelI=on  LabelI=IB_13  Ipu=off  Pbase=100e6  Vbase=500e3  OutputType=Complex  PhasorSimulation=off  PSBequivalent=0
  Bus_ : spsThreePhaseVIMeasurementLib/Three-Phase V-I Measurement  VoltageMeasurement=phase-to-phase  SetLabelV=on  LabelV=V_B13_13  Vpu=off  VpuLL=off  CurrentMeasurement=yes  SetLabelI=on  LabelI=I_B13_13  Ipu=off  Pbase=100e6  Vbase=500e3  OutputType=Complex  PhasorSimulation=off  PSBequivalent=0
  Bus_1 : spsThreePhaseVIMeasurementLib/Three-Phase V-I Measurement  VoltageMeasurement=phase-to-phase  SetLabelV=on  LabelV=V_B13  Vpu=off  VpuLL=off  CurrentMeasurement=yes  SetLabelI=on  LabelI=I_B13  Ipu=off  Pbase=100e6  Vbase=500e3  OutputType=Complex  PhasorSimulation=off  PSBequivalent=0
  Conn1 : PMIOPort  Side=Left
  Conn2 : PMIOPort  Port=2  Side=Right
  Conn3 : PMIOPort  Port=3  Side=Left
  Conn4 : PMIOPort  Port=4  Side=Right
  Conn5 : PMIOPort  Port=5  Side=Right
  Conn6 : PMIOPort  Port=6  Side=Left
  Conn7 : PMIOPort  Port=7  Side=Right
  Conn8 : PMIOPort  Port=8  Side=Right
  Conn9 : PMIOPort  Port=9  Side=Right
  Conn10 : PMIOPort  Port=10  Side=Right
  Conn11 : PMIOPort  Port=11  Side=Right
  Conn12 : PMIOPort  Port=12  Side=Right
  connections:
  Bus_1/LConn1 -- Bus_/LConn3 -- Conn6/RConn1 -- Bus/LConn1
  Conn3/RConn1 -- Bus/LConn2 -- Bus_1/LConn2 -- Bus_/LConn2
  Bus_/RConn2 -- Conn8/RConn1
  Bus/RConn2 -- Conn4/RConn1
  Bus_1/LConn3 -- Bus_/LConn1 -- Conn1/RConn1 -- Bus/LConn3
  Bus_/RConn1 -- Conn7/RConn1
  Bus_/RConn3 -- Conn9/RConn1
  Conn10/RConn1 -- Bus_1/RConn1
  Conn11/RConn1 -- Bus_1/RConn2
  Conn12/RConn1 -- Bus_1/RConn3
  Conn5/RConn1 -- Bus/RConn1
  Conn2/RConn1 -- Bus/RConn3

== system Rooms_integrated_bus13/Power Grid/Bus_14 ==
  Bus : spsThreePhaseVIMeasurementLib/Three-Phase V-I Measurement  VoltageMeasurement=phase-to-phase  SetLabelV=on  LabelV=VB_14  Vpu=off  VpuLL=off  CurrentMeasurement=yes  SetLabelI=on  LabelI=IB_14  Ipu=off  Pbase=100e6  Vbase=500e3  OutputType=Complex  PhasorSimulation=off  PSBequivalent=0
  Bus_ : spsThreePhaseVIMeasurementLib/Three-Phase V-I Measurement  VoltageMeasurement=phase-to-phase  SetLabelV=on  LabelV=V_B14  Vpu=off  VpuLL=off  CurrentMeasurement=yes  SetLabelI=on  LabelI=I_B14  Ipu=off  Pbase=100e6  Vbase=500e3  OutputType=Complex  PhasorSimulation=off  PSBequivalent=0
  Conn1 : PMIOPort  Side=Left
  Conn2 : PMIOPort  Port=2  Side=Right
  Conn3 : PMIOPort  Port=3  Side=Left
  Conn4 : PMIOPort  Port=4  Side=Right
  Conn5 : PMIOPort  Port=5  Side=Right
  Conn6 : PMIOPort  Port=6  Side=Left
  Conn7 : PMIOPort  Port=7  Side=Right
  Conn8 : PMIOPort  Port=8  Side=Right
  Conn9 : PMIOPort  Port=9  Side=Right
  connections:
  Conn1/RConn1 -- Bus_/LConn3 -- Bus/LConn1
  Conn3/RConn1 -- Bus_/LConn2 -- Bus/LConn2
  Bus_/RConn2 -- Conn8/RConn1
  Bus/RConn2 -- Conn4/RConn1
  Bus/LConn3 -- Bus_/LConn1 -- Conn6/RConn1
  Bus/RConn1 -- Conn2/RConn1
  Bus/RConn3 -- Conn5/RConn1
  Conn7/RConn1 -- Bus_/RConn3
  Conn9/RConn1 -- Bus_/RConn1

== system Rooms_integrated_bus13/Power Grid/Bus_2 ==
  Bus : spsThreePhaseVIMeasurementLib/Three-Phase V-I Measurement  VoltageMeasurement=phase-to-phase  SetLabelV=on  LabelV=VB_2  Vpu=off  VpuLL=off  CurrentMeasurement=yes  SetLabelI=on  LabelI=IB_2  Ipu=off  Pbase=100e6  Vbase=500e3  OutputType=Complex  PhasorSimulation=off  PSBequivalent=0
  Bus_ : spsThreePhaseVIMeasurementLib/Three-Phase V-I Measurement  VoltageMeasurement=phase-to-phase  SetLabelV=on  LabelV=V_B22  Vpu=off  VpuLL=off  CurrentMeasurement=yes  SetLabelI=on  LabelI=I_B22  Ipu=off  Pbase=100e6  Vbase=500e3  OutputType=Complex  PhasorSimulation=off  PSBequivalent=0
  Bus_1 : spsThreePhaseVIMeasurementLib/Three-Phase V-I Measurement  VoltageMeasurement=phase-to-phase  SetLabelV=on  LabelV=V_B2  Vpu=off  VpuLL=off  CurrentMeasurement=yes  SetLabelI=on  LabelI=I_B2  Ipu=off  Pbase=100e6  Vbase=500e3  OutputType=Complex  PhasorSimulation=off  PSBequivalent=0
  Conn1 : PMIOPort  Side=Left
  Conn2 : PMIOPort  Port=2  Side=Right
  Conn3 : PMIOPort  Port=3  Side=Left
  Conn4 : PMIOPort  Port=4  Side=Right
  Conn5 : PMIOPort  Port=5  Side=Right
  Conn6 : PMIOPort  Port=6  Side=Left
  Conn7 : PMIOPort  Port=7  Side=Right
  Conn8 : PMIOPort  Port=8  Side=Right
  Conn9 : PMIOPort  Port=9  Side=Right
  Conn10 : PMIOPort  Port=10  Side=Right
  Conn11 : PMIOPort  Port=11  Side=Right
  Conn12 : PMIOPort  Port=12  Side=Right
  Conn13 : PMIOPort  Port=13  Side=Left
  Conn14 : PMIOPort  Port=14  Side=Left
  Conn15 : PMIOPort  Port=15  Side=Left
  Conn16 : PMIOPort  Port=16  Side=Left
  Conn17 : PMIOPort  Port=17  Side=Left
  Conn18 : PMIOPort  Port=18  Side=Left
  connections:
  Bus_1/LConn1 -- Conn18/RConn1 -- Bus_/LConn3 -- Conn13/RConn1 -- Bus/LConn1 -- Conn6/RConn1
  Conn3/RConn1 -- Bus/LConn2 -- Conn17/RConn1 -- Bus_1/LConn2 -- Conn14/RConn1 -- Bus_/LConn2
  Bus_/RConn2 -- Conn8/RConn1
  Bus/RConn2 -- Conn4/RConn1
  Bus_1/LConn3 -- Conn16/RConn1 -- Conn15/RConn1 -- Bus_/LConn1 -- Conn1/RConn1 -- Bus/LConn3
  Bus_/RConn1 -- Conn7/RConn1
  Bus_/RConn3 -- Conn9/RConn1
  Conn10/RConn1 -- Bus_1/RConn1
  Conn11/RConn1 -- Bus_1/RConn2
  Conn12/RConn1 -- Bus_1/RConn3
  Conn5/RConn1 -- Bus/RConn1
  Conn2/RConn1 -- Bus/RConn3

== system Rooms_integrated_bus13/Power Grid/Bus_3 ==
  Bus : spsThreePhaseVIMeasurementLib/Three-Phase V-I Measurement  VoltageMeasurement=phase-to-phase  SetLabelV=on  LabelV=VB_3  Vpu=off  VpuLL=off  CurrentMeasurement=yes  SetLabelI=on  LabelI=IB_3  Ipu=off  Pbase=100e6  Vbase=500e3  OutputType=Complex  PhasorSimulation=off  PSBequivalent=0
  Bus_ : spsThreePhaseVIMeasurementLib/Three-Phase V-I Measurement  VoltageMeasurement=phase-to-phase  SetLabelV=on  LabelV=V_B33  Vpu=off  VpuLL=off  CurrentMeasurement=yes  SetLabelI=on  LabelI=I_B33  Ipu=off  Pbase=100e6  Vbase=500e3  OutputType=Complex  PhasorSimulation=off  PSBequivalent=0
  Bus_1 : spsThreePhaseVIMeasurementLib/Three-Phase V-I Measurement  VoltageMeasurement=phase-to-phase  SetLabelV=on  LabelV=V_B3  Vpu=off  VpuLL=off  CurrentMeasurement=yes  SetLabelI=on  LabelI=I_B3  Ipu=off  Pbase=100e6  Vbase=500e3  OutputType=Complex  PhasorSimulation=off  PSBequivalent=0
  Conn1 : PMIOPort  Side=Left
  Conn2 : PMIOPort  Port=2  Side=Right
  Conn3 : PMIOPort  Port=3  Side=Left
  Conn4 : PMIOPort  Port=4  Side=Right
  Conn5 : PMIOPort  Port=5  Side=Right
  Conn6 : PMIOPort  Port=6  Side=Left
  Conn7 : PMIOPort  Port=7  Side=Right
  Conn8 : PMIOPort  Port=8  Side=Right
  Conn9 : PMIOPort  Port=9  Side=Right
  Conn10 : PMIOPort  Port=10  Side=Right
  Conn11 : PMIOPort  Port=11  Side=Right
  Conn12 : PMIOPort  Port=12  Side=Right
  connections:
  Conn11/RConn1 -- Bus_1/RConn2
  Bus_/RConn3 -- Conn9/RConn1
  Bus_/RConn1 -- Conn7/RConn1
  Bus_1/LConn3 -- Bus_/LConn1 -- Conn1/RConn1 -- Bus/LConn3
  Bus/RConn2 -- Conn4/RConn1
  Bus_/RConn2 -- Conn8/RConn1
  Bus_1/LConn2 -- Bus_/LConn2 -- Bus/LConn2 -- Conn3/RConn1
  Bus_/LConn3 -- Bus_1/LConn1 -- Conn6/RConn1 -- Bus/LConn1
  Conn10/RConn1 -- Bus_1/RConn3
  Conn12/RConn1 -- Bus_1/RConn1
  Conn2/RConn1 -- Bus/RConn3
  Conn5/RConn1 -- Bus/RConn1

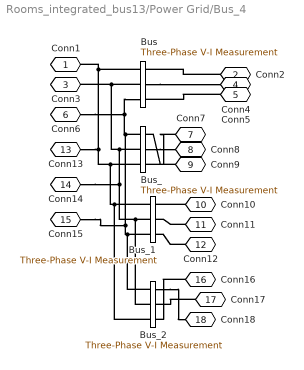
== system Rooms_integrated_bus13/Power Grid/Bus_4 ==
  Bus : spsThreePhaseVIMeasurementLib/Three-Phase V-I Measurement  VoltageMeasurement=phase-to-phase  SetLabelV=on  LabelV=VB_4  Vpu=off  VpuLL=off  CurrentMeasurement=yes  SetLabelI=on  LabelI=IB_4  Ipu=off  Pbase=100e6  Vbase=500e3  OutputType=Complex  PhasorSimulation=off  PSBequivalent=0
  Bus_ : spsThreePhaseVIMeasurementLib/Three-Phase V-I Measurement  VoltageMeasurement=phase-to-phase  SetLabelV=on  LabelV=V_B44  Vpu=off  VpuLL=off  CurrentMeasurement=yes  SetLabelI=on  LabelI=I_B44  Ipu=off  Pbase=100e6  Vbase=500e3  OutputType=Complex  PhasorSimulation=off  PSBequivalent=0
  Bus_1 : spsThreePhaseVIMeasurementLib/Three-Phase V-I Measurement  VoltageMeasurement=phase-to-phase  SetLabelV=on  LabelV=V_B4  Vpu=off  VpuLL=off  CurrentMeasurement=yes  SetLabelI=on  LabelI=I_B4  Ipu=off  Pbase=100e6  Vbase=500e3  OutputType=Complex  PhasorSimulation=off  PSBequivalent=0
  Bus_2 : spsThreePhaseVIMeasurementLib/Three-Phase V-I Measurement  VoltageMeasurement=phase-to-phase  SetLabelV=on  LabelV=V_B4_4  Vpu=off  VpuLL=off  CurrentMeasurement=yes  SetLabelI=on  LabelI=I_B4_4  Ipu=off  Pbase=100e6  Vbase=500e3  OutputType=Complex  PhasorSimulation=off  PSBequivalent=0
  Conn1 : PMIOPort  Side=Left
  Conn2 : PMIOPort  Port=2  Side=Right
  Conn3 : PMIOPort  Port=3  Side=Left
  Conn4 : PMIOPort  Port=4  Side=Right
  Conn5 : PMIOPort  Port=5  Side=Right
  Conn6 : PMIOPort  Port=6  Side=Left
  Conn7 : PMIOPort  Port=7  Side=Right
  Conn8 : PMIOPort  Port=8  Side=Right
  Conn9 : PMIOPort  Port=9  Side=Right
  Conn10 : PMIOPort  Port=10  Side=Right
  Conn11 : PMIOPort  Port=11  Side=Right
  Conn12 : PMIOPort  Port=12  Side=Right
  Conn13 : PMIOPort  Port=13  Side=Left
  Conn14 : PMIOPort  Port=14  Side=Left
  Conn15 : PMIOPort  Port=15  Side=Left
  Conn16 : PMIOPort  Port=16  Side=Right
  Conn17 : PMIOPort  Port=17  Side=Right
  Conn18 : PMIOPort  Port=18  Side=Right
  connections:
  Bus/LConn1 -- Conn1/RConn1 -- Bus_2/LConn3 -- Bus_1/LConn1 -- Bus_/LConn3 -- Conn13/RConn1
  Conn3/RConn1 -- Bus/LConn2 -- Bus_/LConn2 -- Bus_2/LConn2 -- Bus_1/LConn2 -- Conn14/RConn1
  Bus_/RConn2 -- Conn8/RConn1
  Bus/RConn2 -- Conn4/RConn1
  Bus/LConn3 -- Conn6/RConn1 -- Bus_/LConn1 -- Bus_2/LConn1 -- Bus_1/LConn3 -- Conn15/RConn1
  Conn10/RConn1 -- Bus_1/RConn1
  Conn11/RConn1 -- Bus_1/RConn2
  Conn12/RConn1 -- Bus_1/RConn3
  Conn9/RConn1 -- Bus_/RConn1
  Conn7/RConn1 -- Bus_/RConn3
  Conn5/RConn1 -- Bus/RConn3
  Conn2/RConn1 -- Bus/RConn1
  Conn17/RConn1 -- Bus_2/RConn2
  Conn16/RConn1 -- Bus_2/RConn3
  Bus_2/RConn1 -- Conn18/RConn1

== system Rooms_integrated_bus13/Power Grid/Bus_5 ==
  Bus : spsThreePhaseVIMeasurementLib/Three-Phase V-I Measurement  VoltageMeasurement=phase-to-phase  SetLabelV=on  LabelV=VB_5  Vpu=off  VpuLL=off  CurrentMeasurement=yes  SetLabelI=on  LabelI=IB_5  Ipu=off  Pbase=100e6  Vbase=500e3  OutputType=Complex  PhasorSimulation=off  PSBequivalent=0
  Bus_ : spsThreePhaseVIMeasurementLib/Three-Phase V-I Measurement  VoltageMeasurement=phase-to-phase  SetLabelV=on  LabelV=V_B55  Vpu=off  VpuLL=off  CurrentMeasurement=yes  SetLabelI=on  LabelI=I_B55  Ipu=off  Pbase=100e6  Vbase=500e3  OutputType=Complex  PhasorSimulation=off  PSBequivalent=0
  Bus_1 : spsThreePhaseVIMeasurementLib/Three-Phase V-I Measurement  VoltageMeasurement=phase-to-phase  SetLabelV=on  LabelV=V_B5  Vpu=off  VpuLL=off  CurrentMeasurement=yes  SetLabelI=on  LabelI=I_B5  Ipu=off  Pbase=100e6  Vbase=500e3  OutputType=Complex  PhasorSimulation=off  PSBequivalent=0
  Conn1 : PMIOPort  Side=Left
  Conn2 : PMIOPort  Port=2  Side=Right
  Conn3 : PMIOPort  Port=3  Side=Left
  Conn4 : PMIOPort  Port=4  Side=Right
  Conn5 : PMIOPort  Port=5  Side=Right
  Conn6 : PMIOPort  Port=6  Side=Left
  Conn7 : PMIOPort  Port=7  Side=Right
  Conn8 : PMIOPort  Port=8  Side=Right
  Conn9 : PMIOPort  Port=9  Side=Right
  Conn10 : PMIOPort  Port=10  Side=Right
  Conn11 : PMIOPort  Port=11  Side=Right
  Conn12 : PMIOPort  Port=12  Side=Right
  Conn13 : PMIOPort  Port=13  Side=Left
  Conn14 : PMIOPort  Port=14  Side=Left
  Conn15 : PMIOPort  Port=15  Side=Left
  connections:
  Conn12/RConn1 -- Bus_1/RConn3
  Conn11/RConn1 -- Bus_1/RConn2
  Conn10/RConn1 -- Bus_1/RConn1
  Bus_1/LConn3 -- Conn13/RConn1 -- Bus_/LConn1 -- Conn6/RConn1 -- Bus/LConn3
  Bus/RConn2 -- Conn4/RConn1
  Bus_/RConn2 -- Conn8/RConn1
  Conn14/RConn1 -- Bus_1/LConn2 -- Bus_/LConn2 -- Bus/LConn2 -- Conn3/RConn1
  Bus_/LConn3 -- Bus_1/LConn1 -- Conn1/RConn1 -- Bus/LConn1 -- Conn15/RConn1
  Conn7/RConn1 -- Bus_/RConn3
  Conn9/RConn1 -- Bus_/RConn1
  Conn5/RConn1 -- Bus/RConn1
  Conn2/RConn1 -- Bus/RConn3

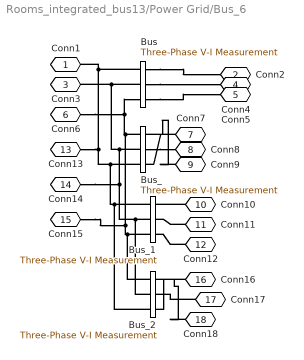
== system Rooms_integrated_bus13/Power Grid/Bus_6 ==
  Bus : spsThreePhaseVIMeasurementLib/Three-Phase V-I Measurement  VoltageMeasurement=phase-to-phase  SetLabelV=on  LabelV=VB_6  Vpu=off  VpuLL=off  CurrentMeasurement=yes  SetLabelI=on  LabelI=IB_6  Ipu=off  Pbase=100e6  Vbase=500e3  OutputType=Complex  PhasorSimulation=off  PSBequivalent=0
  Bus_ : spsThreePhaseVIMeasurementLib/Three-Phase V-I Measurement  VoltageMeasurement=phase-to-phase  SetLabelV=on  LabelV=V_B66  Vpu=off  VpuLL=off  CurrentMeasurement=yes  SetLabelI=on  LabelI=I_B66  Ipu=off  Pbase=100e6  Vbase=500e3  OutputType=Complex  PhasorSimulation=off  PSBequivalent=0
  Bus_1 : spsThreePhaseVIMeasurementLib/Three-Phase V-I Measurement  VoltageMeasurement=phase-to-phase  SetLabelV=on  LabelV=V_B6  Vpu=off  VpuLL=off  CurrentMeasurement=yes  SetLabelI=on  LabelI=I_B6  Ipu=off  Pbase=100e6  Vbase=500e3  OutputType=Complex  PhasorSimulation=off  PSBequivalent=0
  Bus_2 : spsThreePhaseVIMeasurementLib/Three-Phase V-I Measurement  VoltageMeasurement=phase-to-phase  SetLabelV=on  LabelV=V_B6_6  Vpu=off  VpuLL=off  CurrentMeasurement=yes  SetLabelI=on  LabelI=I_B6_6  Ipu=off  Pbase=100e6  Vbase=500e3  OutputType=Complex  PhasorSimulation=off  PSBequivalent=0
  Conn1 : PMIOPort  Side=Left
  Conn2 : PMIOPort  Port=2  Side=Right
  Conn3 : PMIOPort  Port=3  Side=Left
  Conn4 : PMIOPort  Port=4  Side=Right
  Conn5 : PMIOPort  Port=5  Side=Right
  Conn6 : PMIOPort  Port=6  Side=Left
  Conn7 : PMIOPort  Port=7  Side=Right
  Conn8 : PMIOPort  Port=8  Side=Right
  Conn9 : PMIOPort  Port=9  Side=Right
  Conn10 : PMIOPort  Port=10  Side=Right
  Conn11 : PMIOPort  Port=11  Side=Right
  Conn12 : PMIOPort  Port=12  Side=Right
  Conn13 : PMIOPort  Port=13  Side=Left
  Conn14 : PMIOPort  Port=14  Side=Left
  Conn15 : PMIOPort  Port=15  Side=Left
  Conn16 : PMIOPort  Port=16  Side=Right
  Conn17 : PMIOPort  Port=17  Side=Right
  Conn18 : PMIOPort  Port=18  Side=Right
  connections:
  Conn17/RConn1 -- Bus_2/RConn2
  Conn12/RConn1 -- Bus_1/RConn3
  Conn11/RConn1 -- Bus_1/RConn2
  Conn10/RConn1 -- Bus_1/RConn1
  Bus/RConn3 -- Conn5/RConn1
  Bus/RConn1 -- Conn2/RConn1
  Bus_2/LConn1 -- Bus_1/LConn3 -- Conn15/RConn1 -- Bus_/LConn1 -- Conn6/RConn1 -- Bus/LConn3
  Bus/RConn2 -- Conn4/RConn1
  Bus_/RConn2 -- Conn8/RConn1
  Bus_2/LConn2 -- Bus_1/LConn2 -- Conn14/RConn1 -- Bus_/LConn2 -- Bus/LConn2 -- Conn3/RConn1
  Bus_2/LConn3 -- Bus_1/LConn1 -- Bus_/LConn3 -- Conn13/RConn1 -- Conn1/RConn1 -- Bus/LConn1
  Conn7/RConn1 -- Bus_/RConn3
  Conn9/RConn1 -- Bus_/RConn1
  Conn16/RConn1 -- Bus_2/RConn3
  Conn18/RConn1 -- Bus_2/RConn1

== system Rooms_integrated_bus13/Power Grid/Bus_7 ==
  Bus : spsThreePhaseVIMeasurementLib/Three-Phase V-I Measurement  VoltageMeasurement=phase-to-phase  SetLabelV=on  LabelV=VB_7  Vpu=off  VpuLL=off  CurrentMeasurement=yes  SetLabelI=on  LabelI=IB_7  Ipu=off  Pbase=100e6  Vbase=500e3  OutputType=Complex  PhasorSimulation=off  PSBequivalent=0
  Bus_ : spsThreePhaseVIMeasurementLib/Three-Phase V-I Measurement  VoltageMeasurement=phase-to-phase  SetLabelV=on  LabelV=V_B7  Vpu=off  VpuLL=off  CurrentMeasurement=yes  SetLabelI=on  LabelI=I_B7  Ipu=off  Pbase=100e6  Vbase=500e3  OutputType=Complex  PhasorSimulation=off  PSBequivalent=0
  Conn1 : PMIOPort  Side=Left
  Conn2 : PMIOPort  Port=2  Side=Right
  Conn3 : PMIOPort  Port=3  Side=Left
  Conn4 : PMIOPort  Port=4  Side=Right
  Conn5 : PMIOPort  Port=5  Side=Right
  Conn6 : PMIOPort  Port=6  Side=Left
  Conn7 : PMIOPort  Port=7  Side=Right
  Conn8 : PMIOPort  Port=8  Side=Right
  Conn9 : PMIOPort  Port=9  Side=Right
  connections:
  Bus_/LConn3 -- Bus/LConn1 -- Conn6/RConn1
  Conn3/RConn1 -- Bus_/LConn2 -- Bus/LConn2
  Bus_/RConn2 -- Conn8/RConn1
  Bus/RConn2 -- Conn4/RConn1
  Bus_/LConn1 -- Conn1/RConn1 -- Bus/LConn3
  Bus_/RConn1 -- Conn7/RConn1
  Bus_/RConn3 -- Conn9/RConn1
  Conn2/RConn1 -- Bus/RConn3
  Conn5/RConn1 -- Bus/RConn1
